simulink model "hw1_pendulum"  (R2017a)
settings: Solver=ode45  StartTime=0.0  StopTime=10.0  RelTol=1e-3  EnableMultiTasking=on
InitFcn:
  | M = 1;
  | b = 1;
  | R = 1;
  | g = 9.81;
libraries: simulink x1
settings Model: Creator=edward  LastModifiedBy=edward
settings DataIOCC: LimitDataPoints=on  SaveFormat=Array
settings OptimizationCC: LifeSpan=inf
settings DebuggingCC: UnderspecifiedInitializationDetection=Classic  MergeDetectMultiDrivingBlocksExec=none  SolverPrmCheckMsg=warning  SFUnexpectedBacktrackingDiag=warning  SFNoUnconditionalDefaultTransitionDiag=warning  SFExecutionAtInitializationDiag=none
settings HardwareCC: ProdBitPerPointer=32  ProdBitPerSizeT=32  ProdBitPerPtrDiffT=32  ProdLargestAtomicFloat=None  ProdIntDivRoundTo=Undefined  ProdEndianess=Unspecified  ProdWordSize=32  ProdHWDeviceType=32-bit Generic
settings ModelReferenceCC: PropagateSignalLabelsOutOfModel=off
settings GRTTargetCC: TargetLangStandard=C89/C90 (ANSI)  GeneratePreprocessorConditionals=Disable all
settings ConfigComp: CovMetricSettings=dw  CovHtmlReporting=on  CovSaveCumulativeToWorkspaceVar=on  CovSaveSingleToWorkspaceVar=on  CovExternalEMLEnable=off

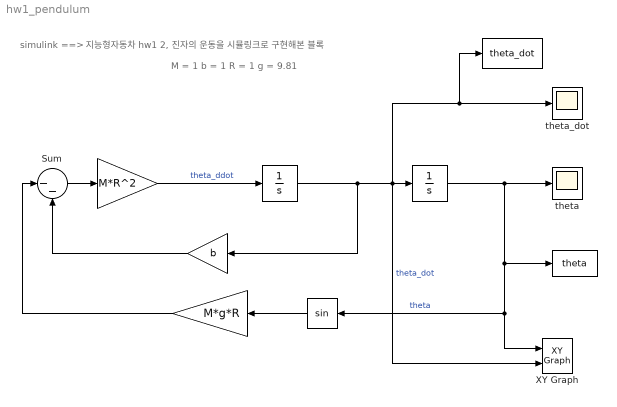
== system hw1_pendulum ==
  note: simulink ==> 지능형자동차 hw1 2, 진자의 운동을 시뮬링크로 구현해본 블록
  note: M = 1
      | b = 1
      | R = 1
      | g = 9.81
  " " : Gain  Gain=b
  "  " : Gain  Gain=M*g*R
  "   " : Trigonometry
  "    " : Gain  Gain=M*R^2
  "     " : Integrator
  "      " : Integrator  InitialCondition=pi/3
  "        " : ToWorkspace  VariableName=theta_dot  SaveFormat=Timeseries  SampleTime=-1
  "         " : ToWorkspace  VariableName=theta  SaveFormat=Timeseries  SampleTime=-1
  Sum : Sum  Inputs=|--
  XY Graph : simulink/Sinks/XY Graph  xmin=-1  xmax=1  ymin=-1  ymax=1  st=-1
  theta : Scope
  theta_dot : Scope
  wires:
  Sum/1 -> "    "/1
  "    "/1 -> "     "/1  "theta_ddot"
  "     "/1 -> XY Graph/2, "        "/1, theta_dot/1, "      "/1, " "/1  "theta_dot"
  " "/1 -> Sum/2
  "      "/1 -> XY Graph/1, "   "/1, "         "/1, theta/1  "theta"
  "  "/1 -> Sum/1
  "   "/1 -> "  "/1
